simulink model "control_assemblyRules_4docking"  (R2020a)
settings: Solver=FixedStepAuto  StartTime=0.0  StopTime=60  FixedStep=0.025  RelTol=1e-3  EnableMultiTasking=on
InitFcn:
  | global clientID;
  | clientID=-1;
  | 
  | global R_t;
  | global A_t;
  | global P_t;
  | global H;
  | global Q;
  | global N;
  | 
  | R_t=eye(3);
  | A_t=eye(3)*0;
  | P_t=eye(3)*0.001;
  | H=eye(3);
  | Q=eye(3);
  | N=eye(3);
values from neighbouring files (symbols this model uses):
  W = eye(8)    [kumar_controller.m]
  X = reshape(X, size(A_t))    [RiccatiCov.m]
undefined symbols (not defined in the file or in its folder): Y, Z
libraries: robotlib x21, dspindex x3, simulink_extras x1
settings Model: SimulationMode=external  Creator=Kleber Cabral  LastModifiedBy=Kleber Cabral
settings SolverCC: AutoInsertRateTranBlk=on
settings DataIOCC: SaveFormat=Array  ReturnWorkspaceOutputs=off
settings OptimizationCC: EnhancedBackFolding=on  PassReuseOutputArgsAs=Individual arguments  ZeroExternalMemoryAtStartup=off  ZeroInternalMemoryAtStartup=off  MaxStackSize=64  OptimizeBlockOrder=speed  DifferentSizesBufferReuse=on  OptimizationCustomize=off  EfficientTunableParamExpr=on
settings DebuggingCC: SolverPrmCheckMsg=warning  ParameterTunabilityLossMsg=error  SFUnexpectedBacktrackingDiag=warning  SFNoUnconditionalDefaultTransitionDiag=warning  ArithmeticOperatorsInVariantConditions=warning
settings HardwareCC: ProdBitPerPointer=32  ProdBitPerSizeT=32  ProdBitPerPtrDiffT=32  ProdLargestAtomicFloat=None  ProdIntDivRoundTo=Undefined  ProdEndianess=Unspecified  ProdWordSize=32  ProdHWDeviceType=Generic->Unspecified (assume 32-bit Generic)  UseEmbeddedCoderFeatures=off
settings ModelReferenceCC: PropagateSignalLabelsOutOfModel=off
settings SFSimCC: SimUseLocalCustomCode=off  MATLABDynamicMemAlloc=off  CustomCodeUndefinedFunction=UseInterfaceOnly
settings RTWCC: SystemTargetFile=ert.tlc  HardwareBoard=Robot Operating System (ROS)  TemplateMakefile=ert_default_tmf  RTWUseLocalCustomCode=off  Toolchain=Catkin  TargetLang=C++
settings CodeAppCC: ForceParamTrailComments=on  IgnoreCustomStorageClasses=off  OperatorAnnotations=on  SimulinkDataObjDesc=on  SFDataObjDesc=on  InsertBlockDesc=on
settings ERTTargetCC: SupportNonInlinedSFcns=on
settings ConfigComp: CovMetricSettings=dw  CovHtmlReporting=on  CovSaveCumulativeToWorkspaceVar=on  CovSaveSingleToWorkspaceVar=on  CovExternalEMLEnable=off  CovSFcnEnable=off

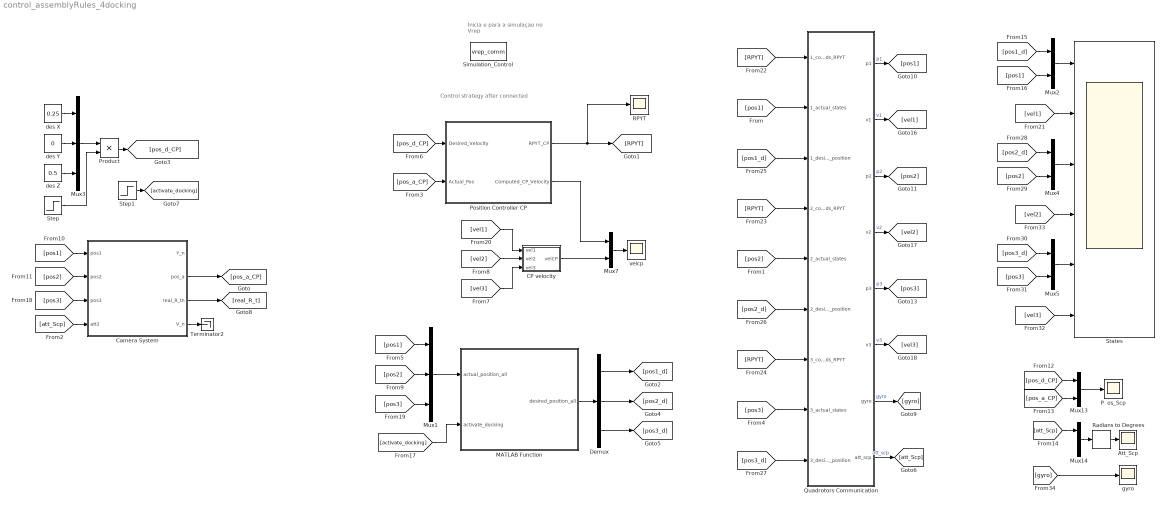
== system control_assemblyRules_4docking ==
  note: Control strategy after connected
  note: Inicia e para a simulaçao no Vrep
  Att_Scp : Scope
  CP velocity : Subsystem
  Camera System : Subsystem
  Demux : Demux  Outputs=3
  MATLAB Function : MATLAB Function  TreatAsAtomicUnit=on
  Mux1 : Mux  Inputs=3
  Mux{2,4..5,7,13..14} (6 alike) : Mux  Inputs=2
  Mux3 : Mux  Inputs=3
  P  os_Scp : Scope
  Position Controller CP : Subsystem
  Product : Product
  Quadrotors Communication : Subsystem
  RPYT : Scope
  Radians to Degrees : simulink_extras/Transformations/Radians to Degrees
  Simulation_Control : S-Function  FunctionName=vrep_comm  SFunctionDeploymentMode=off  EnableBusSupport=off
  States : Scope  NumInputPorts=6
  Step : Step  Time=2  SampleTime=0
  Step1 : Step  Time=10  SampleTime=0
  Terminator2 : Terminator
  des X : Constant  Value=0.25
  des Y : Constant  Value=0
  des Z : Constant  Value=0.5
  gyro : Scope
  velcp : Scope
  wires:
  des X/1 -> Mux3/1
  des Y/1 -> Mux3/2
  des Z/1 -> Mux3/3
  [pos1] -> Camera System/1(pos1)
  [pos2] -> Camera System/2(pos2)
  [pos1] -> Quadrotors Communication/2(1_actual_states)
  [pos2] -> Quadrotors Communication/5(2_actual_states)
  Camera System/2(pos_a) -> [pos_a_CP]
  [att_Scp] -> Camera System/4(att2)
  Mux3/1 -> Product/1
  Step/1 -> Product/2
  Product/1 -> [pos_d_CP]
  Mux13/1 -> P  os_Scp/1
  [pos_d_CP] -> Mux13/1
  [pos_a_CP] -> Mux13/2
  [att_Scp] -> Mux14/1
  Camera System/3(real_R_tn) -> [real_R_t]
  Camera System/4(V_n) -> Terminator2/1
  Quadrotors Communication/1(p1) -> [pos1]  "p1"
  Quadrotors Communication/2(v1) -> [vel1]  "v1"
  Quadrotors Communication/3(p2) -> [pos2]  "p2"
  Quadrotors Communication/4(v2) -> [vel2]  "v2"
  Quadrotors Communication/7(gyro) -> [gyro]  "gyro"
  Quadrotors Communication/8(att_scp) -> [att_Scp]  "att_scp"
  Quadrotors Communication/5(p3) -> [pos3]  "p3"
  [pos3] -> Camera System/3(pos3)
  Quadrotors Communication/6(v3) -> [vel3]  "v3"
  [pos3] -> Quadrotors Communication/8(3_actual_states)
  Radians to Degrees/1 -> Att_Scp/1
  Mux14/1 -> Radians to Degrees/1
  CP velocity/1(velCP) -> Mux7/2
  [vel2] -> CP velocity/2(vel2)
  [vel1] -> CP velocity/1(vel1)
  [vel3] -> CP velocity/3(vel3)
  Mux7/1 -> velcp/1
  [RPYT] -> Quadrotors Communication/1(1_commands_RPYT)
  [pos_d_CP] -> Position Controller CP/1(Desired_Velocity)
  [pos_a_CP] -> Position Controller CP/2(Actual_Pos)
  Position Controller CP/2(Computed_CP_Velocity) -> Mux7/1
  [pos1] -> Mux1/1
  [pos2] -> Mux1/2
  [pos3] -> Mux1/3
  Mux1/1 -> MATLAB Function/1(actual_position_all)
  Position Controller CP/1(RPYT_CP) -> RPYT/1, [RPYT]
  MATLAB Function/1(desired_position_all) -> Demux/1
  Demux/3 -> [pos3_d]
  [RPYT] -> Quadrotors Communication/4(2_commands_RPYT)
  [RPYT] -> Quadrotors Communication/7(3_commands_RPYT)
  [pos1_d] -> Quadrotors Communication/3(1_desired_position)
  [pos2_d] -> Quadrotors Communication/6(2_desired_position)
  [pos3_d] -> Quadrotors Communication/9(3_desired_position)
  Mux2/1 -> States/1
  [pos1_d] -> Mux2/1
  Demux/1 -> [pos1_d]
  Step1/1 -> [activate_docking]
  Demux/2 -> [pos2_d]
  [activate_docking] -> MATLAB Function/2(activate_docking)
  [pos1] -> Mux2/2
  [vel1] -> States/2
  [pos2] -> Mux4/2
  [pos2_d] -> Mux4/1
  [pos3_d] -> Mux5/1
  [pos3] -> Mux5/2
  Mux4/1 -> States/3
  Mux5/1 -> States/5
  [vel3] -> States/6
  [vel2] -> States/4
  [gyro] -> gyro/1

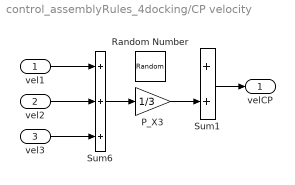
== system control_assemblyRules_4docking/CP velocity ==
  vel1 : Inport
  vel2 : Inport  Port=2
  vel3 : Inport  Port=3
  P_X3 : Gain  Gain=1/3
  Random Number : RandomNumber  Variance=0.02*0.02
  Sum1 : Sum
  Sum6 : Sum  Inputs=+++
  velCP : Outport  VectorParamsAs1DForOutWhenUnconnected=off
  wires:
  vel2/1 -> Sum6/2
  vel3/1 -> Sum6/3
  vel1/1 -> Sum6/1
  P_X3/1 -> Sum1/2
  Sum1/1 -> velCP/1
  Sum6/1 -> P_X3/1

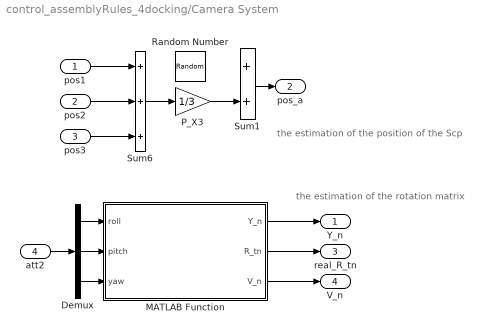
== system control_assemblyRules_4docking/Camera System ==
  note: the estimation of the rotation matrix
  note: the estimation of the position of the Scp
  pos1 : Inport
  pos2 : Inport  Port=2
  pos3 : Inport  Port=3
  att2 : Inport  Port=4
  Demux : Demux  Outputs=3
  MATLAB Function : MATLAB Function  TreatAsAtomicUnit=on
  P_X3 : Gain  Gain=1/3
  Random Number : RandomNumber  Variance=0.02*0.02
  Sum1 : Sum
  Sum6 : Sum  Inputs=+++
  Y_n : Outport  VectorParamsAs1DForOutWhenUnconnected=off
  pos_a : Outport  Port=2  VectorParamsAs1DForOutWhenUnconnected=off
  real_R_tn : Outport  Port=3  VectorParamsAs1DForOutWhenUnconnected=off
  V_n : Outport  Port=4  VectorParamsAs1DForOutWhenUnconnected=off
  wires:
  pos1/1 -> Sum6/1
  pos2/1 -> Sum6/2
  Sum6/1 -> P_X3/1
  Sum1/1 -> pos_a/1
  att2/1 -> Demux/1
  Demux/3 -> MATLAB Function/3(yaw)
  Demux/2 -> MATLAB Function/2(pitch)
  Demux/1 -> MATLAB Function/1(roll)
  MATLAB Function/1(Y_n) -> Y_n/1
  MATLAB Function/2(R_tn) -> real_R_tn/1
  MATLAB Function/3(V_n) -> V_n/1
  pos3/1 -> Sum6/3
  P_X3/1 -> Sum1/2

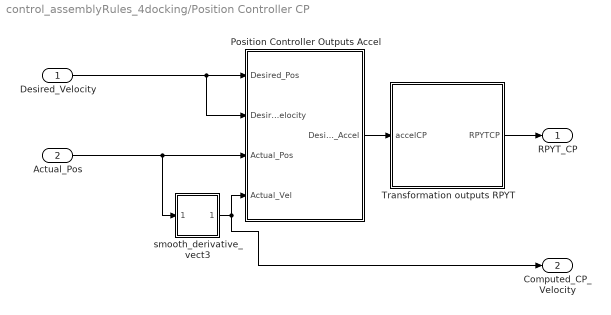
== system control_assemblyRules_4docking/Position Controller CP ==
  Desired_Velocity : Inport
  Actual_Pos : Inport  Port=2
  Position Controller Outputs Accel : Subsystem
  Transformation outputs RPYT : Subsystem
  smooth_derivative_vect3 : Subsystem
  RPYT_CP : Outport
  Computed_CP_Velocity : Outport  Port=2
  wires:
  Position Controller Outputs Accel/1(Desired_Accel) -> Transformation outputs RPYT/1(accelCP)
  Transformation outputs RPYT/1(RPYTCP) -> RPYT_CP/1
  Desired_Velocity/1 -> Position Controller Outputs Accel/2(Desired_Velocity), Position Controller Outputs Accel/1(Desired_Pos)
  smooth_derivative_vect3/1(Out1) -> Position Controller Outputs Accel/4(Actual_Vel), Computed_CP_Velocity/1
  Actual_Pos/1 -> Position Controller Outputs Accel/3(Actual_Pos), smooth_derivative_vect3/1(In1)

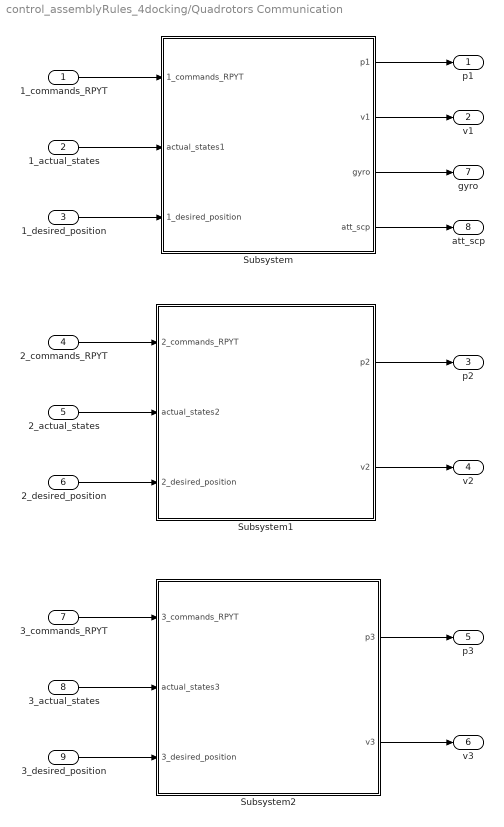
== system control_assemblyRules_4docking/Quadrotors Communication ==
  1_commands_RPYT : Inport
  1_actual_states : Inport  Port=2
  1_desired_position : Inport  Port=3
  2_commands_RPYT : Inport  Port=4
  2_actual_states : Inport  Port=5
  2_desired_position : Inport  Port=6
  3_commands_RPYT : Inport  Port=7
  3_actual_states : Inport  Port=8
  3_desired_position : Inport  Port=9
  Subsystem : Subsystem
  Subsystem1 : Subsystem
  Subsystem2 : Subsystem
  p1 : Outport  VectorParamsAs1DForOutWhenUnconnected=off
  v1 : Outport  Port=2  VectorParamsAs1DForOutWhenUnconnected=off
  p2 : Outport  Port=3  VectorParamsAs1DForOutWhenUnconnected=off
  v2 : Outport  Port=4  VectorParamsAs1DForOutWhenUnconnected=off
  p3 : Outport  Port=5  VectorParamsAs1DForOutWhenUnconnected=off
  v3 : Outport  Port=6  VectorParamsAs1DForOutWhenUnconnected=off
  gyro : Outport  Port=7  VectorParamsAs1DForOutWhenUnconnected=off
  att_scp : Outport  Port=8  VectorParamsAs1DForOutWhenUnconnected=off
  wires:
  1_commands_RPYT/1 -> Subsystem/1(1_commands_RPYT)
  1_actual_states/1 -> Subsystem/2(actual_states1)
  Subsystem/1(p1) -> p1/1
  Subsystem/2(v1) -> v1/1
  Subsystem/3(gyro) -> gyro/1
  Subsystem/4(att_scp) -> att_scp/1
  2_commands_RPYT/1 -> Subsystem1/1(2_commands_RPYT)
  2_actual_states/1 -> Subsystem1/2(actual_states2)
  Subsystem1/1(p2) -> p2/1
  Subsystem1/2(v2) -> v2/1
  3_commands_RPYT/1 -> Subsystem2/1(3_commands_RPYT)
  3_actual_states/1 -> Subsystem2/2(actual_states3)
  Subsystem2/1(p3) -> p3/1
  Subsystem2/2(v3) -> v3/1
  1_desired_position/1 -> Subsystem/3(1_desired_position)
  2_desired_position/1 -> Subsystem1/3(2_desired_position)
  3_desired_position/1 -> Subsystem2/3(3_desired_position)

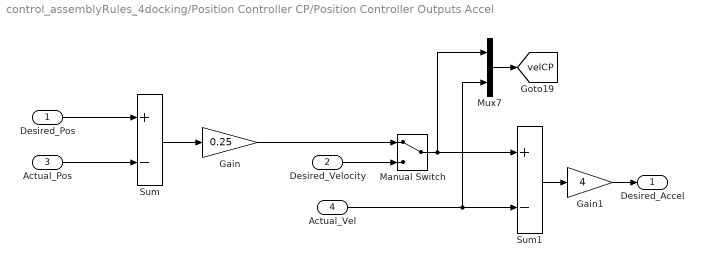
== system control_assemblyRules_4docking/Position Controller CP/Position Controller Outputs Accel ==
  Desired_Pos : Inport
  Desired_Velocity : Inport  Port=2
  Actual_Pos : Inport  Port=3
  Actual_Vel : Inport  Port=4
  Gain : Gain  Gain=0.25
  Gain1 : Gain  Gain=4
  Manual Switch : ManualSwitch
  Mux7 : Mux  Inputs=2
  Sum : Sum  Inputs=+-
  Sum1 : Sum  Inputs=+-
  Desired_Accel : Outport  VectorParamsAs1DForOutWhenUnconnected=off
  tag scope: velCP=global
  wires:
  Sum/1 -> Gain/1
  Desired_Pos/1 -> Sum/1
  Sum1/1 -> Gain1/1
  Actual_Vel/1 -> Mux7/2, Sum1/2
  Gain1/1 -> Desired_Accel/1
  Actual_Pos/1 -> Sum/2
  Desired_Velocity/1 -> Manual Switch/2
  Gain/1 -> Manual Switch/1
  Manual Switch/1 -> Sum1/1, Mux7/1
  Mux7/1 -> [velCP]

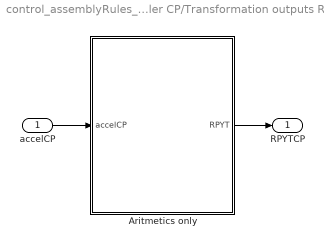
== system control_assemblyRules_4docking/Position Controller CP/Transformation outputs RPYT ==
  accelCP : Inport
  Aritmetics only : MATLAB Function  TreatAsAtomicUnit=on
  RPYTCP : Outport  VectorParamsAs1DForOutWhenUnconnected=off
  wires:
  Aritmetics only/1(RPYT) -> RPYTCP/1
  accelCP/1 -> Aritmetics only/1(accelCP)

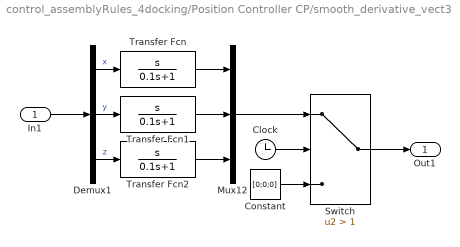
== system control_assemblyRules_4docking/Position Controller CP/smooth_derivative_vect3 ==
  In1 : Inport
  Clock : Clock
  Constant : Constant  Value=[0;0;0]
  Demux1 : Demux  Outputs=3
  Mux12 : Mux  Inputs=3
  Switch : Switch  Criteria=u2 > Threshold  Threshold=1
  Transfer Fcn : TransferFcn  Numerator=[1 0]  Denominator=[0.1 1]
  Transfer Fcn1 : TransferFcn  Numerator=[1 0]  Denominator=[0.1 1]
  Transfer Fcn2 : TransferFcn  Numerator=[1 0]  Denominator=[0.1 1]
  Out1 : Outport  VectorParamsAs1DForOutWhenUnconnected=off
  wires:
  Transfer Fcn/1 -> Mux12/1
  Transfer Fcn2/1 -> Mux12/3
  Transfer Fcn1/1 -> Mux12/2
  Switch/1 -> Out1/1
  Demux1/1 -> Transfer Fcn/1  "x"
  Demux1/2 -> Transfer Fcn1/1  "y"
  Demux1/3 -> Transfer Fcn2/1  "z"
  In1/1 -> Demux1/1
  Constant/1 -> Switch/3
  Clock/1 -> Switch/2
  Mux12/1 -> Switch/1

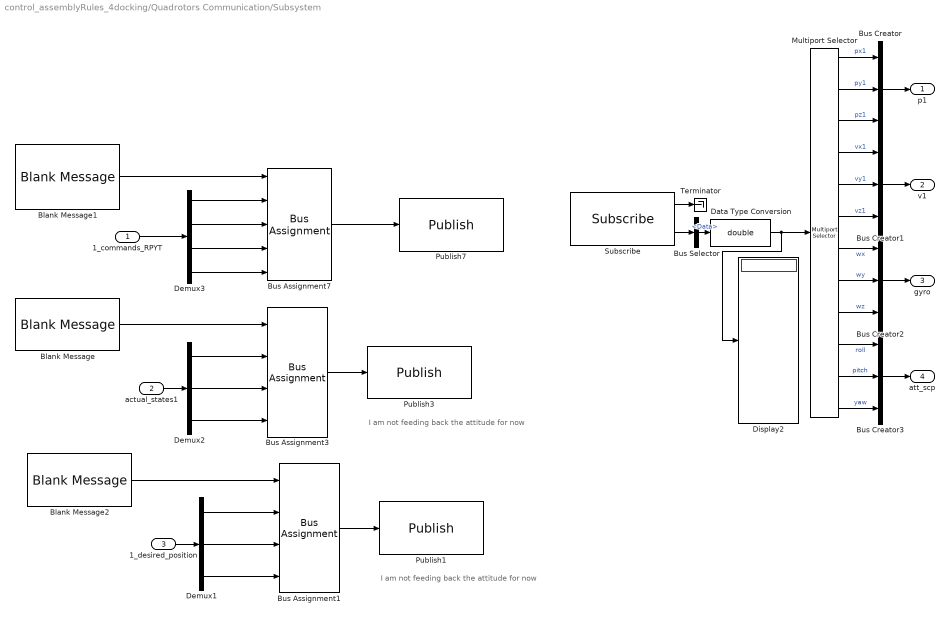
== system control_assemblyRules_4docking/Quadrotors Communication/Subsystem ==
  note: I am not feeding back the attitude for now
  note: I am not feeding back the attitude for now
  1_commands_RPYT : Inport
  actual_states1 : Inport  Port=2
  1_desired_position : Inport  Port=3
  Blank Message : robotlib/Blank Message  messageClass=Message  entityType=geometry_msgs/Vector3  messageType=geometry_msgs/Vector3  SampleTime=inf
  Blank Message1 : robotlib/Blank Message  messageClass=Message  entityType=geometry_msgs/Quaternion  messageType=geometry_msgs/Quaternion  SampleTime=inf
  Blank Message2 : robotlib/Blank Message  messageClass=Message  entityType=geometry_msgs/Vector3  messageType=geometry_msgs/Vector3  SampleTime=inf
  Bus Assignment1 : BusAssignment  DialogController=Simulink.DDGSource_BusAssignment  AssignedSignals=X,Y,Z
  Bus Assignment3 : BusAssignment  DialogController=Simulink.DDGSource_BusAssignment  AssignedSignals=X,Y,Z
  Bus Assignment7 : BusAssignment  DialogController=Simulink.DDGSource_BusAssignment  AssignedSignals=X,Y,Z,W
  Bus Creator{,1..3} (4 alike) : BusCreator  Inputs=3
  Bus Selector : BusSelector  OutputSignals=Data
  Data Type Conversion : DataTypeConversion  OutDataTypeStr=double
  Demux1 : Demux  Outputs=3
  Demux2 : Demux  Outputs=3
  Demux3 : Demux
  Display2 : Display
      settings: Decimation=3
  Multiport Selector : dspindex/Multiport Selector  rowsOrCols=Rows  idxCellArray={1,2,3,4,5,6,7,8,9,10,11,12}  idxErrMode=Clip Index
  Publish1 : robotlib/Publish  topicSource=Select from ROS network  topic=/desired_waypoint_0  messageType=geometry_msgs/Vector3  messageQueueLength=105
  Publish3 : robotlib/Publish  topicSource=Select from ROS network  topic=/actual_states_0  messageType=geometry_msgs/Vector3  messageQueueLength=105
  Publish7 : robotlib/Publish  topicSource=Specify your own  topic=/commands_attitude_0  messageType=geometry_msgs/Quaternion  messageQueueLength=105
  Subscribe : robotlib/Subscribe  topicSource=Select from ROS network  topic=/quadrotor_states_0  messageType=std_msgs/Float32MultiArray  sampleTime=-1  messageQueueLength=51
  Terminator : Terminator
  p1 : Outport  VectorParamsAs1DForOutWhenUnconnected=off
  v1 : Outport  Port=2  VectorParamsAs1DForOutWhenUnconnected=off
  gyro : Outport  Port=3  VectorParamsAs1DForOutWhenUnconnected=off
  att_scp : Outport  Port=4  VectorParamsAs1DForOutWhenUnconnected=off
  wires:
  Multiport Selector/2 -> Bus Creator/2  "py1"
  Multiport Selector/12 -> Bus Creator3/3  "yaw"
  Demux3/4 -> Bus Assignment7/5
  Demux3/1 -> Bus Assignment7/2
  Blank Message/1 -> Bus Assignment3/1
  Blank Message1/1 -> Bus Assignment7/1
  Multiport Selector/8 -> Bus Creator2/2  "wy"
  Bus Assignment3/1 -> Publish3/1
  Data Type Conversion/1 -> Display2/1, Multiport Selector/1
  Bus Creator2/1 -> gyro/1
  Demux2/1 -> Bus Assignment3/2
  Multiport Selector/3 -> Bus Creator/3  "pz1"
  Multiport Selector/11 -> Bus Creator3/2  "pitch"
  Bus Creator1/1 -> v1/1
  Multiport Selector/7 -> Bus Creator2/1  "wx"
  Demux3/2 -> Bus Assignment7/3
  Multiport Selector/6 -> Bus Creator1/3  "vz1"
  Bus Creator3/1 -> att_scp/1
  Multiport Selector/9 -> Bus Creator2/3  "wz"
  Multiport Selector/1 -> Bus Creator/1  "px1"
  Demux2/3 -> Bus Assignment3/4
  1_commands_RPYT/1 -> Demux3/1
  Subscribe/2 -> Bus Selector/1
  Demux3/3 -> Bus Assignment7/4
  Bus Creator/1 -> p1/1
  Multiport Selector/10 -> Bus Creator3/1  "roll"
  Demux2/2 -> Bus Assignment3/3
  Multiport Selector/5 -> Bus Creator1/2  "vy1"
  Multiport Selector/4 -> Bus Creator1/1  "vx1"
  Subscribe/1 -> Terminator/1
  actual_states1/1 -> Demux2/1
  Bus Selector/1 -> Data Type Conversion/1  "<Data>"
  1_desired_position/1 -> Demux1/1
  Demux1/2 -> Bus Assignment1/3
  Demux1/3 -> Bus Assignment1/4
  Demux1/1 -> Bus Assignment1/2
  Bus Assignment1/1 -> Publish1/1
  Blank Message2/1 -> Bus Assignment1/1
  Bus Assignment7/1 -> Publish7/1

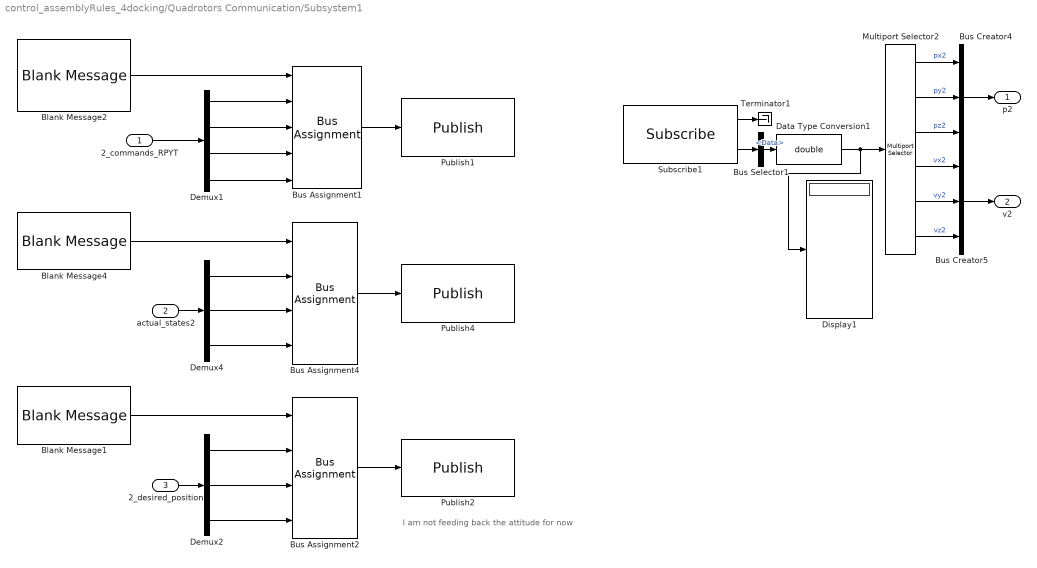
== system control_assemblyRules_4docking/Quadrotors Communication/Subsystem1 ==
  note: I am not feeding back the attitude for now
  2_commands_RPYT : Inport
  actual_states2 : Inport  Port=2
  2_desired_position : Inport  Port=3
  Blank Message1 : robotlib/Blank Message  messageClass=Message  entityType=geometry_msgs/Vector3  messageType=geometry_msgs/Vector3  SampleTime=inf
  Blank Message2 : robotlib/Blank Message  messageClass=Message  entityType=geometry_msgs/Quaternion  messageType=geometry_msgs/Quaternion  SampleTime=inf
  Blank Message4 : robotlib/Blank Message  messageClass=Message  entityType=geometry_msgs/Vector3  messageType=geometry_msgs/Vector3  SampleTime=inf
  Bus Assignment1 : BusAssignment  DialogController=Simulink.DDGSource_BusAssignment  AssignedSignals=X,Y,Z,W
  Bus Assignment2 : BusAssignment  DialogController=Simulink.DDGSource_BusAssignment  AssignedSignals=X,Y,Z
  Bus Assignment4 : BusAssignment  DialogController=Simulink.DDGSource_BusAssignment  AssignedSignals=X,Y,Z
  Bus Creator4 : BusCreator  Inputs=3
  Bus Creator5 : BusCreator  Inputs=3
  Bus Selector1 : BusSelector  OutputSignals=Data
  Data Type Conversion1 : DataTypeConversion  OutDataTypeStr=double
  Demux1 : Demux
  Demux2 : Demux  Outputs=3
  Demux4 : Demux  Outputs=3
  Display1 : Display
      settings: Decimation=3
  Multiport Selector2 : dspindex/Multiport Selector  rowsOrCols=Rows  idxCellArray={1,2,3,4,5,6}  idxErrMode=Clip Index
  Publish1 : robotlib/Publish  topicSource=Select from ROS network  topic=/commands_attitude_1  messageType=geometry_msgs/Quaternion  messageQueueLength=105
  Publish2 : robotlib/Publish  topicSource=Select from ROS network  topic=/desired_waypoint_1  messageType=geometry_msgs/Vector3  messageQueueLength=105
  Publish4 : robotlib/Publish  topicSource=Select from ROS network  topic=/actual_states_1  messageType=geometry_msgs/Vector3  messageQueueLength=105
  Subscribe1 : robotlib/Subscribe  topicSource=Select from ROS network  topic=/quadrotor_states_1  messageType=std_msgs/Float32MultiArray  sampleTime=-1  messageQueueLength=51
  Terminator1 : Terminator
  p2 : Outport  VectorParamsAs1DForOutWhenUnconnected=off
  v2 : Outport  Port=2  VectorParamsAs1DForOutWhenUnconnected=off
  wires:
  Multiport Selector2/1 -> Bus Creator4/1  "px2"
  actual_states2/1 -> Demux4/1
  Bus Assignment4/1 -> Publish4/1
  Multiport Selector2/2 -> Bus Creator4/2  "py2"
  Blank Message2/1 -> Bus Assignment1/1
  Bus Assignment1/1 -> Publish1/1
  Demux4/1 -> Bus Assignment4/2
  Subscribe1/1 -> Terminator1/1
  Bus Creator4/1 -> p2/1
  Demux1/3 -> Bus Assignment1/4
  Demux1/1 -> Bus Assignment1/2
  Demux4/3 -> Bus Assignment4/4
  Bus Creator5/1 -> v2/1
  Subscribe1/2 -> Bus Selector1/1
  Multiport Selector2/5 -> Bus Creator5/2  "vy2"
  2_commands_RPYT/1 -> Demux1/1
  Bus Selector1/1 -> Data Type Conversion1/1  "<Data>"
  Multiport Selector2/6 -> Bus Creator5/3  "vz2"
  Demux1/4 -> Bus Assignment1/5
  Multiport Selector2/4 -> Bus Creator5/1  "vx2"
  Demux4/2 -> Bus Assignment4/3
  Demux1/2 -> Bus Assignment1/3
  Multiport Selector2/3 -> Bus Creator4/3  "pz2"
  Blank Message4/1 -> Bus Assignment4/1
  Data Type Conversion1/1 -> Display1/1, Multiport Selector2/1
  Demux2/2 -> Bus Assignment2/3
  Demux2/1 -> Bus Assignment2/2
  Bus Assignment2/1 -> Publish2/1
  2_desired_position/1 -> Demux2/1
  Blank Message1/1 -> Bus Assignment2/1
  Demux2/3 -> Bus Assignment2/4

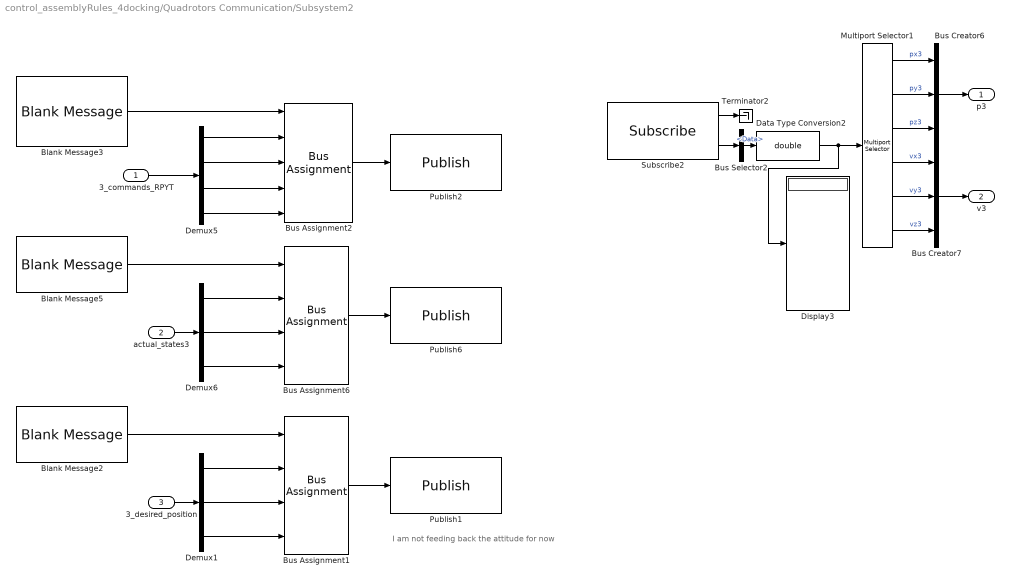
== system control_assemblyRules_4docking/Quadrotors Communication/Subsystem2 ==
  note: I am not feeding back the attitude for now
  3_commands_RPYT : Inport
  actual_states3 : Inport  Port=2
  3_desired_position : Inport  Port=3
  Blank Message2 : robotlib/Blank Message  messageClass=Message  entityType=geometry_msgs/Vector3  messageType=geometry_msgs/Vector3  SampleTime=inf
  Blank Message3 : robotlib/Blank Message  messageClass=Message  entityType=geometry_msgs/Quaternion  messageType=geometry_msgs/Quaternion  SampleTime=inf
  Blank Message5 : robotlib/Blank Message  messageClass=Message  entityType=geometry_msgs/Vector3  messageType=geometry_msgs/Vector3  SampleTime=inf
  Bus Assignment1 : BusAssignment  DialogController=Simulink.DDGSource_BusAssignment  AssignedSignals=X,Y,Z
  Bus Assignment2 : BusAssignment  DialogController=Simulink.DDGSource_BusAssignment  AssignedSignals=X,Y,Z,W
  Bus Assignment6 : BusAssignment  DialogController=Simulink.DDGSource_BusAssignment  AssignedSignals=X,Y,Z
  Bus Creator6 : BusCreator  Inputs=3
  Bus Creator7 : BusCreator  Inputs=3
  Bus Selector2 : BusSelector  OutputSignals=Data
  Data Type Conversion2 : DataTypeConversion  OutDataTypeStr=double
  Demux1 : Demux  Outputs=3
  Demux5 : Demux
  Demux6 : Demux  Outputs=3
  Display3 : Display
      settings: Decimation=3
  Multiport Selector1 : dspindex/Multiport Selector  rowsOrCols=Rows  idxCellArray={1,2,3,4,5,6}  idxErrMode=Clip Index
  Publish1 : robotlib/Publish  topicSource=Select from ROS network  topic=/desired_waypoint_2  messageType=geometry_msgs/Vector3  messageQueueLength=105
  Publish2 : robotlib/Publish  topicSource=Select from ROS network  topic=/commands_attitude_2  messageType=geometry_msgs/Quaternion  messageQueueLength=105
  Publish6 : robotlib/Publish  topicSource=Select from ROS network  topic=/actual_states_2  messageType=geometry_msgs/Vector3  messageQueueLength=105
  Subscribe2 : robotlib/Subscribe  topicSource=Select from ROS network  topic=/quadrotor_states_2  messageType=std_msgs/Float32MultiArray  sampleTime=-1  messageQueueLength=51
  Terminator2 : Terminator
  p3 : Outport  VectorParamsAs1DForOutWhenUnconnected=off
  v3 : Outport  Port=2  VectorParamsAs1DForOutWhenUnconnected=off
  wires:
  Multiport Selector1/1 -> Bus Creator6/1  "px3"
  Bus Creator6/1 -> p3/1
  actual_states3/1 -> Demux6/1
  Demux6/1 -> Bus Assignment6/2
  Multiport Selector1/5 -> Bus Creator7/2  "vy3"
  Demux6/2 -> Bus Assignment6/3
  Bus Assignment2/1 -> Publish2/1
  Bus Creator7/1 -> v3/1
  Multiport Selector1/3 -> Bus Creator6/3  "pz3"
  Subscribe2/1 -> Terminator2/1
  3_commands_RPYT/1 -> Demux5/1
  Demux5/2 -> Bus Assignment2/3
  Data Type Conversion2/1 -> Multiport Selector1/1, Display3/1
  Demux5/4 -> Bus Assignment2/5
  Multiport Selector1/6 -> Bus Creator7/3  "vz3"
  Subscribe2/2 -> Bus Selector2/1
  Multiport Selector1/4 -> Bus Creator7/1  "vx3"
  Blank Message3/1 -> Bus Assignment2/1
  Demux6/3 -> Bus Assignment6/4
  Demux5/1 -> Bus Assignment2/2
  Demux5/3 -> Bus Assignment2/4
  Blank Message5/1 -> Bus Assignment6/1
  Bus Assignment6/1 -> Publish6/1
  Multiport Selector1/2 -> Bus Creator6/2  "py3"
  Bus Selector2/1 -> Data Type Conversion2/1  "<Data>"
  Demux1/2 -> Bus Assignment1/3
  Demux1/1 -> Bus Assignment1/2
  Bus Assignment1/1 -> Publish1/1
  3_desired_position/1 -> Demux1/1
  Blank Message2/1 -> Bus Assignment1/1
  Demux1/3 -> Bus Assignment1/4

== matlab function control_assemblyRules_4docking/MATLAB Function ==
  data: actual_position_all input; desired_position_all output; activate_docking input
function desired_position_all  = Docking_Control(actual_position_all, activate_docking)

    n=3;
    dt=0.025;
    N=3;%length(actual_position_all)/n;
    A=ones(N,N)-eye(N);
    x=reshape(actual_position_all,[n,N]);
    method=1;

    if activate_docking == 0
        desired_position_all=actual_position_all;
        for i=1:N
            desired_position_all(i*n)=0.5;
        end
    else
    
        %Rules for docking
        %% Method 1 - Network Control
        if method==1
            %trying network control based on position only
            for i=1:N
                    posi = x(1:n,i);
            %         veli = x(n+1:n+n,i,k);
                    u = x(1:n,1)*0;

                    for j=1:N
                        posj = x(1:n,j);
                        if i~=j && A(i,j)~=0
                            fprintf('[%d,%d]\n', int32(i),int32(j))
            %                 posj = x(1:n,j);
            %                 velj = x(n+1:n+n,j);
                            u = u + (posi - posj);%+ kv*(veli-velj);
                        end
                    end
                    u=-1*u;
                    x(1:n,i) = posi+dt*u;
            end
            desired_position_all=reshape(x,[1,N*n])';
%             (actual_position_all-desired_position_all)'
        end

        %% Method 2 - Mean
        if method==2
            desired_position_all=[mean(x,2);mean(x,2);mean(x,2)];
%             (actual_position_all-desired_position_all)'
        end
    end
end

== matlab function control_assemblyRules_4docking/Camera System/MATLAB Function ==
  data: roll input; Y_n output; pitch input; yaw input; R_tn output; V_n output
function [Y_n,R_tn,V_n] = EulerAng2RotMat(roll, pitch, yaw)
% a=deg2rad(0);
% b=deg2rad(0);
% c=deg2rad(45);

a=roll;
b=pitch;
c=yaw;

sa=sin(a);ca=cos(a);
sb=sin(b);cb=cos(b);
sc=sin(c);cc=cos(c);
R_tn=[ cc*cb cc*sb*sa-sc*ca cc*sb*ca+sc*sa 
    sc*cb sc*sb*sa+cc*ca sc*sb*ca-cc*sa 
    -sb       cb*sa           cb*ca     ];

%noise of about 1 deg of rotation in each axis
a=deg2rad(randn*2);
b=deg2rad(randn*2);
c=deg2rad(randn*2);
sa=sin(a);ca=cos(a);
sb=sin(b);cb=cos(b);
sc=sin(c);cc=cos(c);
V_n=[ cc*cb cc*sb*sa-sc*ca cc*sb*ca+sc*sa 
    sc*cb sc*sb*sa+cc*ca sc*sb*ca-cc*sa 
    -sb       cb*sa           cb*ca     ];

Y_n = R_tn * V_n;

%R = R *(eye(3)+0.001*randn(3,3));
end

== matlab function control_assemblyRules_4docking/Position Controller CP/Transformation outputs RPYT/Aritmetics only ==
  data: accelCP input; RPYT output
function RPYT   = ACCEL2RPYT(accelCP)
g=9.81;
m=0.0563;
Tcp=m*g+m*accelCP(3);
RPYT=[rad2deg(-accelCP(2)/g);
    rad2deg(accelCP(1)/g);
    rad2deg(0);
    Tcp];
end
